simulink model "Model1"  (R2020b)
settings: Solver=VariableStepAuto  StartTime=0.0  StopTime=10.0  RelTol=1e-3
values from neighbouring files (symbols this model uses):
  b = 50    [S1.m]
  k1 = 50    [S1.m]
  k12 = 100*M2    (= 5000)    [S1.m]
  M1 = 100    [S1.m]
  M2 = 50    [S1.m]
settings Model: Creator=Diwakar Reddy  LastModifiedBy=Diwakar Reddy

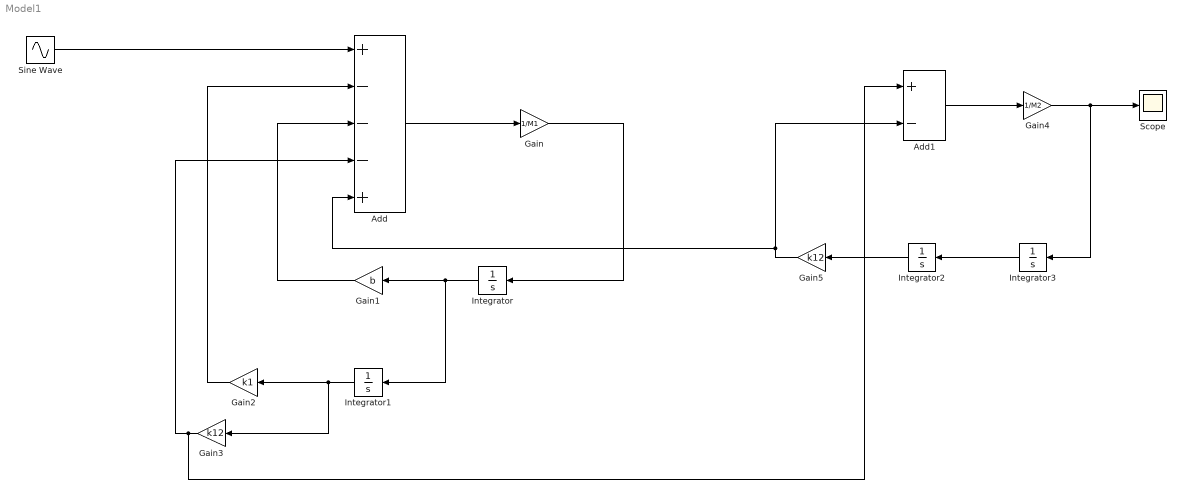
== system Model1 ==
  Add : Sum  Inputs=+---+
  Add1 : Sum  Inputs=+-
  Gain : Gain  Gain=1/M1
  Gain1 : Gain  Gain=b
  Gain2 : Gain  Gain=k1
  Gain3 : Gain  Gain=k12
  Gain4 : Gain  Gain=1/M2
  Gain5 : Gain  Gain=k12
  Integrator{,1..3} (4 alike) : Integrator
  Scope : Scope
  Sine Wave : Sin  Amplitude=2  Frequency=10  SampleTime=0
  wires:
  Add/1 -> Gain/1
  Gain/1 -> Integrator/1
  Integrator/1 -> Integrator1/1, Gain1/1
  Gain1/1 -> Add/3
  Sine Wave/1 -> Add/1
  Integrator1/1 -> Gain3/1, Gain2/1
  Gain2/1 -> Add/2
  Gain3/1 -> Add1/1, Add/4
  Add1/1 -> Gain4/1
  Integrator3/1 -> Integrator2/1
  Integrator2/1 -> Gain5/1
  Gain4/1 -> Scope/1, Integrator3/1
  Gain5/1 -> Add/5, Add1/2
